simulink model "msk_sync"  (Simulink 6.0)
settings: Solver=FixedStepDiscrete  SolverMode=SingleTasking  StartTime=0.0  StopTime=2.0  RelTol=1e-3
PreLoadFcn:
  | warning off MATLAB:dispatcher:InexactMatch;
model workspace: external: M-Code (data not in the file)
undefined symbols (not defined in the file or in its folder): sampPerSymb, slcm, tsym
libraries: dspsrcs4 x9, simulink x5, commsink2 x4, dspsigops x4, commblksprivate x2, dspsigattribs x2, dspstat3 x2, commutil2 x2, commdigbbndcpm2 x2, dspobslib x1, commfilt2 x1, dspmathops x1
CloseFcn:
  | if exist('msk_sync_sigsOut','var'), clear msk_sync_sigsOut; end;
  | warning on MATLAB:dispatcher:InexactMatch;
settings Model: Creator=arodrigu  LastModifiedBy=cvora  ExtModeAutoUpdateStatusClock=off  ProdHWDeviceType=Specified
settings DataIOCC: LimitDataPoints=off  SaveOutput=off  SaveTime=off  SignalLoggingName=msk_sync_sigsOut
settings OptimizationCC: BooleanDataType=off
settings DebuggingCC: CheckExecutionContextPreStartOutputMsg=on  CheckExecutionContextRuntimeOutputMsg=on  SolverPrmCheckMsg=none  InheritedTsInSrcMsg=none
settings HardwareCC: ProdHWDeviceType=Specified
settings ModelReferenceCC: UpdateModelReferenceTargets=IfOutOfDate

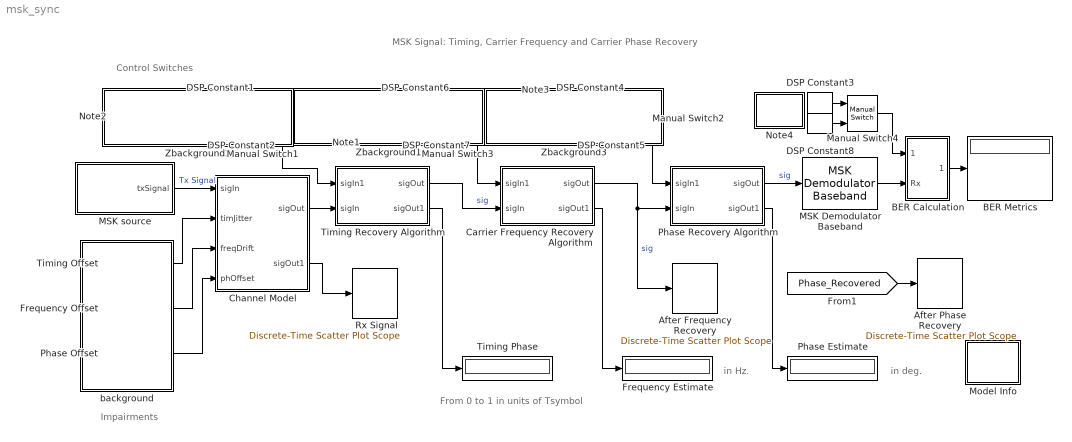
== system msk_sync ==
  note: MSK Signal:
      | Timing, Carrier Frequency and Carrier Phase Recovery
  note: in Hz.
  note: From 0 to 1
      | in units of Tsymbol
  note: in deg.
  note: Control Switches
  note: Impairments
  After Frequency Recovery : commsink2/Discrete-Time Scatter Plot Scope  Tag=ScatterPlot  sampPerSymb=1  offsetEye=0  numTraces=2000  numNewFrames=1000  LineMarkers=.  LineColors=b  fading=on  render=on  AxisGrid=on  xMin=-1.5  xMax=1.5  yMin=-1.5  yMax=1.5  inphaseLabel=In-phase Amplitude  quadratureLabel=Quadrature Amplitude  openScopeAtSimStart=on  FrameNumber=off  FigPos=[435 41 358 358]  figTitle=Scatter Plot  numLinesMax=8  block_type_=scatter
  After Phase Recovery : commsink2/Discrete-Time Scatter Plot Scope  Tag=ScatterPlot  sampPerSymb=1  offsetEye=0  numTraces=2000  numNewFrames=1000  LineMarkers=.  LineColors=b  fading=on  render=on  AxisGrid=on  xMin=-1.5  xMax=1.5  yMin=-1.5  yMax=1.5  inphaseLabel=In-phase Amplitude  quadratureLabel=Quadrature Amplitude  openScopeAtSimStart=on  FrameNumber=off  FigPos=[832 41 358 358]  figTitle=Scatter Plot  numLinesMax=8  block_type_=scatter
  BER Calculation : Subsystem  PropExecContextAcrossSSBoundary=on
      mask Display: disp('BER')
  BER Metrics : Display
  Carrier Frequency Recovery Algorithm : Subsystem  PropExecContextAcrossSSBoundary=on
      mask Type: Carrier Frequency Recovery algorithm
      mask Display: disp('Carrier Freq.\nRecovery')
  Channel Model : Subsystem  PropExecContextAcrossSSBoundary=on
      mask Type: RF Impairments
      mask Display:
      | plot(-10,-10,110, 110,[05 15 10 10 05 10 18 14 13 7.5 13 41 44 47 50 53 57
      | 59 100-[13 7.5 13 14 18 10 5 10 10 15 5]],[70 70 70 85 92 85 79 82 90 88.5
      | 90 90 87 93 87 93 87 90 90 88.5 90 82 79 85 92 85 70 70 70]-30);
  DSP Constant{1,3..4,6} (4 alike) : dspsrcs4/DSP Constant  Value=1  SampleMode=Discrete  discreteOutput=Sample-based (interpret vectors as 1-D)  continuousOutput=Sample-based  sampTime=tsym*1000  framePeriod=tsym*1000  dataType=Inherit from 'Constant value'  isSigned=on  wordLen=16  udDataType=sfix(16)  fracBitsMode=Best precision  numFracBits=15  InterpretAs1D=on  Ts=tsym*1000  FramebasedOutput=off
      settings: AttributesFormatString=\n\n\n\n
  DSP Constant{2,5,7..8} (4 alike) : dspsrcs4/DSP Constant  Value=0  SampleMode=Discrete  discreteOutput=Sample-based (interpret vectors as 1-D)  continuousOutput=Sample-based  sampTime=tsym*1000  framePeriod=tsym*1000  dataType=Inherit from 'Constant value'  isSigned=on  wordLen=16  udDataType=sfix(16)  fracBitsMode=Best precision  numFracBits=15  InterpretAs1D=on  Ts=tsym*1000  FramebasedOutput=off
      settings: AttributesFormatString=\n\n\n\n
  Frequency Estimate : Display
  Frequency Offset : Constant  Value=50
  MSK Demodulator Baseband : commdigbbndcpm2/MSK Demodulator Baseband  outputType=Bit  phaseOffset=0  samplesPerSymbol=1  traceBack=trDepth
  MSK source : Subsystem  PropExecContextAcrossSSBoundary=on
      mask Type: GMSK source
      mask Display: disp('MSK\nSource')
  Manual Switch1 : simulink/Signal Routing/Manual Switch  sw=1  action=0
  Manual Switch2 : simulink/Signal Routing/Manual Switch  sw=1  action=0
  Manual Switch3 : simulink/Signal Routing/Manual Switch  sw=1  action=0
  Manual Switch4 : simulink/Signal Routing/Manual Switch  sw=0  action=0
  Model Info : Subsystem  LoadFcn=slcm LoadBlock;  InitFcn=slcm('UpdateAllCMBlocksInThisModelInit')  PropExecContextAcrossSSBoundary=on  mask(CMBlock){InitialSaveTempField=, InitialBlockCM=None, BlockCM=None, Frame=on, SaveTempField=, DisplayStringWithTags=Info, MaskDisplayString=Info, HorizontalTextAlignment=Center, LeftAlignmentValue=0.5, SourceBlockDiagram=msk_sync, TagMaxNumber=20, CMTag1=, CMTag2=, CMTag3=, CMTag4=, CMTag5=, CMTag6=, CMTag7=, CMTag8=, CMTag9=, CMTag10=, CMTag11=, CMTag12=, CMTag13=, CMTag14=, CMTag15=, CMTag16=, CMTag17=, CMTag18=, CMTag19=, CMTag20=}
      mask help: This block allows revision control information to be displayed within the model.
      settings: CopyFcn=slcm CopyBlock;  DeleteFcn=slcm Cancel;  PostSaveFcn=slcm('UpdateAllCMBlocksInThisModel')  NameChangeFcn=slcm Rename;  OpenFcn=commdemohelp;
      mask Display: text(str2num(LeftAlignmentValue), 0.5, MaskDisplayString, 'HorizontalAlignment', HorizontalTextAlignment)
  Note1 : Subsystem  PropExecContextAcrossSSBoundary=on
      mask Display: disp('Carrier Frequency\nRecovery')
  Note2 : Subsystem  PropExecContextAcrossSSBoundary=on
      mask Display: disp('Timing Phase\nRecovery')
  Note3 : Subsystem  PropExecContextAcrossSSBoundary=on
      mask Display: disp('Phase\nRecovery')
  Note4 : Subsystem  PropExecContextAcrossSSBoundary=on
      mask Display: disp('Reset\nBER')
  Phase Estimate : Display
  Phase Offset : Constant  Value=30
  Phase Recovery Algorithm : Subsystem  PropExecContextAcrossSSBoundary=on
      mask Type: Carrier Frequency Recovery algorithm
      mask Display: disp('Phase\nRecovery')
  Rx Signal : commsink2/Discrete-Time Scatter Plot Scope  Tag=ScatterPlot  sampPerSymb=14  offsetEye=0  numTraces=2000  numNewFrames=1000  LineMarkers=.  LineColors=b  fading=on  render=on  AxisGrid=on  xMin=-1.5  xMax=1.5  yMin=-1.5  yMax=1.5  inphaseLabel=In-phase Amplitude  quadratureLabel=Quadrature Amplitude  openScopeAtSimStart=on  FrameNumber=off  FigPos=[38 41 358 358]  figTitle=Scatter Plot  numLinesMax=8  block_type_=scatter
  Timing Offset : Constant  Value=0.2
  Timing Phase : Display
  Timing Recovery Algorithm : Subsystem  PropExecContextAcrossSSBoundary=on
      mask Type: Timing recovery algorithm.
      mask Display: disp('Timing\nRecovery');
  Zbackground1 : Subsystem  PropExecContextAcrossSSBoundary=on
      mask Display: disp('')
  Zbackground2 : Subsystem  PropExecContextAcrossSSBoundary=on
      mask Display: disp('')
  Zbackground3 : Subsystem  PropExecContextAcrossSSBoundary=on
      mask Display: disp('')
  background : Subsystem  PropExecContextAcrossSSBoundary=on
      mask Display: disp('')
  wires:
  Carrier Frequency Recovery Algorithm/1(sigOut) -> Phase Recovery Algorithm/2(sigIn), After Frequency Recovery/1  "sig"
  MSK source/1(txSignal) -> Channel Model/1(sigIn)  "Tx Signal"
  Channel Model/1(sigOut) -> Timing Recovery Algorithm/2(sigIn)
  Manual Switch1/1 -> Timing Recovery Algorithm/1(sigIn1)
  Timing Recovery Algorithm/1(sigOut) -> Carrier Frequency Recovery Algorithm/2(sigIn)  "sig"
  Manual Switch3/1 -> Carrier Frequency Recovery Algorithm/1(sigIn1)
  Timing Offset/1 -> Channel Model/2(timJitter)
  Frequency Offset/1 -> Channel Model/3(freqDrift)
  Timing Recovery Algorithm/2(sigOut1) -> Timing Phase/1
  Carrier Frequency Recovery Algorithm/2(sigOut1) -> Frequency Estimate/1
  Phase Recovery Algorithm/2(sigOut1) -> Phase Estimate/1
  Phase Offset/1 -> Channel Model/4(phOffset)
  Phase Recovery Algorithm/1(sigOut) -> MSK Demodulator Baseband/1  "sig"
  MSK Demodulator Baseband/1 -> BER Calculation/2(Rx)
  BER Calculation/1(Out1) -> BER Metrics/1
  Channel Model/2(sigOut1) -> Rx Signal/1
  Manual Switch4/1 -> BER Calculation/1(Rst)
  [Phase_Recovered] -> After Phase Recovery/1
  Manual Switch2/1 -> Phase Recovery Algorithm/1(sigIn1)
  DSP Constant4/1 -> Manual Switch2/1
  DSP Constant5/1 -> Manual Switch2/2
  DSP Constant6/1 -> Manual Switch3/1
  DSP Constant7/1 -> Manual Switch3/2
  DSP Constant1/1 -> Manual Switch1/1
  DSP Constant2/1 -> Manual Switch1/2
  DSP Constant3/1 -> Manual Switch4/1
  DSP Constant8/1 -> Manual Switch4/2

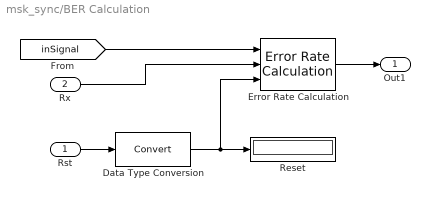
== system msk_sync/BER Calculation ==
  Rst : Inport  LatchInput=off
  Rx : Inport  Port=2  LatchInput=off
  Data Type Conversion : DataTypeConversion  OutDataTypeMode=double
  Error Rate Calculation : commsink2/Error Rate Calculation  N=trDepth+2 % Traceback Depth + Delay due to Timing Recovery  st_delay=0  cp_mode=Entire frame  subframe=[]  PMode=Port  WsName=ErrorVec  RsMode2=on  stop=off  numErr=100  maxBits=1e6
  Reset : Display
  Out1 : Outport
  wires:
  Error Rate Calculation/1 -> Out1/1
  Rst/1 -> Data Type Conversion/1
  Data Type Conversion/1 -> Reset/1, Error Rate Calculation/3
  Rx/1 -> Error Rate Calculation/2
  [inSignal] -> Error Rate Calculation/1

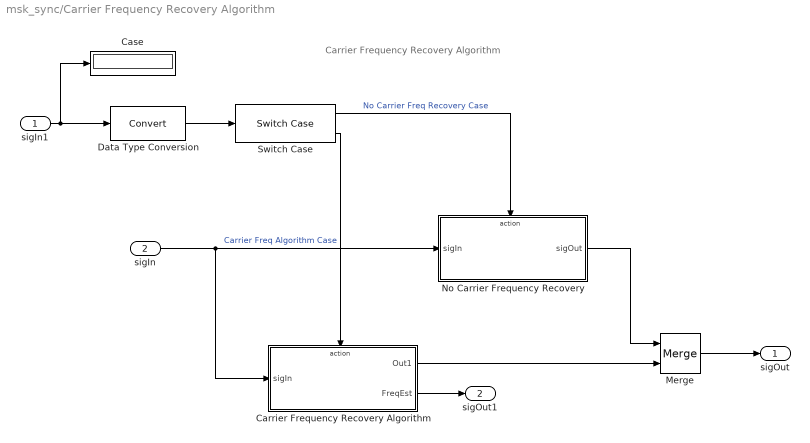
== system msk_sync/Carrier Frequency Recovery Algorithm ==
  note: Carrier Frequency Recovery Algorithm
  sigIn1 : Inport  LatchInput=off
  sigIn : Inport  Port=2  LatchInput=off
  Carrier Frequency Recovery Algorithm : Subsystem  TreatAsAtomicUnit=on  PropExecContextAcrossSSBoundary=on
  Case : Display
  Data Type Conversion : DataTypeConversion  OutDataTypeMode=double
  Merge : Merge
  No Carrier Frequency Recovery : Subsystem  TreatAsAtomicUnit=on  PropExecContextAcrossSSBoundary=on
  Switch Case : SwitchCase  CaseConditions={0,1}  CaseShowDefault=off
  sigOut : Outport
  sigOut1 : Outport  Port=2
  wires:
  sigIn/1 -> No Carrier Frequency Recovery/1(sigIn), Carrier Frequency Recovery Algorithm/1(sigIn)
  Merge/1 -> sigOut/1
  Switch Case/2 -> Carrier Frequency Recovery Algorithm/Action  "Carrier Freq Algorithm Case"
  Switch Case/1 -> No Carrier Frequency Recovery/Action  "No Carrier Freq Recovery Case"
  No Carrier Frequency Recovery/1(sigOut) -> Merge/1
  Carrier Frequency Recovery Algorithm/1(Out1) -> Merge/2
  Carrier Frequency Recovery Algorithm/2(FreqEst) -> sigOut1/1
  sigIn1/1 -> Data Type Conversion/1, Case/1
  Data Type Conversion/1 -> Switch Case/1

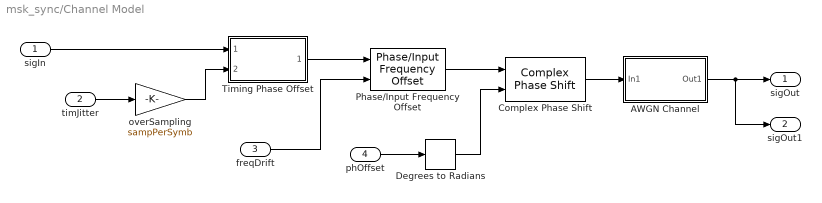
== system msk_sync/Channel Model ==
  sigIn : Inport  LatchInput=off
  timJitter : Inport  Port=2  LatchInput=off
  freqDrift : Inport  Port=3  LatchInput=off
  phOffset : Inport  Port=4  LatchInput=off
  AWGN Channel : Subsystem  AncestorBlock=commchan2/AWGN Channel  PropExecContextAcrossSSBoundary=on  mask(AWGN Channel){seed=67, noiseMode=Signal to noise ratio  (Eb/No), EbNodB=60, EsNodB=10, SNRdB=10, bitsPerSym=1, Ps=1, Tsym=tsym, variance=1}
      mask prompts: seed "Initial seed:"; noiseMode "Mode:"; EbNodB "Eb/No (dB):"; EsNodB "Es/No (dB):"; SNRdB "SNR (dB):"; bitsPerSym "Number of bits per symbol:"; Ps "Input signal power (watts):"; Tsym "Symbol period (s):"
      mask help:
      | Add white Gaussian noise to the input signal. The input and output signals can be real or complex. This block supports multichannel input and output signals as well as frame-based processing.
      |
      | When using either of the variance modes with complex inputs, the variance values are equally divided among the real and imaginary components of the input signal.
      mask init:
      | [mode,s]=commblkawgnchan2(gcb,'init');
      | if ~isempty(s.status) error(s.status); end
      mask Help: helpview(commbhelp)
      mask StyleString: edit,popup(Signal to noise ratio  (Eb/No)|Signal to noise ratio  (Es/No)|Signal to noise ratio  (SNR)|Variance from mask|Variance from port),edit,edit,edit,edit,edit,edit,edit
      mask CallbackString: |commblkawgnchan2(gcb,'Mode');|||||||
      mask Display:
      | plot(-10,-10,110, 110,[05 15 10 10 05 10 18 14 13 7.5 13 41 44 47 50 53 57
      | 59 100-[13 7.5 13 14 18 10 5 10 10 15 5]],[70 70 70 85 92 85 79 82 90 88.5
      | 90 90 87 93 87 93 87 90 90 88.5 90 82 79 85 92 85 70 70 70]);
      | disp('AWGN');
      | port_label('input',s.i1,s.i1s);
      | port_label('input',s.i2,s.i2s);
      | port_label('output',s.o1,s.o1s);
  Complex Phase Shift : commutil2/Complex Phase Shift
  Degrees to Radians : simulink_extras/Transformations/Degrees to Radians
  Phase/Input Frequency Offset : commblksprivate/Phase//Input Frequency Offset  phaseOffset=0
  Timing Phase Offset : Subsystem  PropExecContextAcrossSSBoundary=on
      mask Display: disp('Timing Phase\nOffset')
  overSampling : Gain  Gain=sampPerSymb  SaturateOnIntegerOverflow=on
  sigOut : Outport
  sigOut1 : Outport  Port=2
  wires:
  AWGN Channel/1(Out1) -> sigOut/1, sigOut1/1
  sigIn/1 -> Timing Phase Offset/1(InSignal)
  timJitter/1 -> overSampling/1
  Timing Phase Offset/1(OutSignal) -> Phase/Input Frequency Offset/1
  overSampling/1 -> Timing Phase Offset/2(phOffset)
  freqDrift/1 -> Phase/Input Frequency Offset/2
  Phase/Input Frequency Offset/1 -> Complex Phase Shift/1
  Complex Phase Shift/1 -> AWGN Channel/1(In1)
  Degrees to Radians/1 -> Complex Phase Shift/2
  phOffset/1 -> Degrees to Radians/1

== system msk_sync/MSK source ==
  note: in bps.
  Bernoulli Binary Generator : commrandsrc2/Bernoulli Binary Generator  P=0.5  seed=61  Ts=tsym  frameBased=on  sampPerFrame=1000  orient=off
  Compute Bit Rate : Subsystem  PropExecContextAcrossSSBoundary=on  mask(Compute bit rate of signal ){overSamp=sampPerSymb}
      mask prompts: overSamp "Oversampling factor:"
      mask help: Bit rate calculation based on probed sample time and a specified number of bits per sample.
      mask Display: disp('Compute\nBit Rate')
  MSK Modulator Baseband : commdigbbndcpm2/MSK Modulator Baseband  inputType=Bit  phaseOffset=0  samplesPerSymbol=sampPerSymb
  bit rate : Display
  txSignal : Outport
  tag scope: inSignal=global
  wires:
  Bernoulli Binary Generator/1 -> [inSignal], MSK Modulator Baseband/1
  MSK Modulator Baseband/1 -> Compute Bit Rate/1(sig), txSignal/1
  Compute Bit Rate/1(rate) -> bit rate/1

== system msk_sync/Model Info ==
  EmptySubsystem : Subsystem  PropExecContextAcrossSSBoundary=on

== system msk_sync/Note1 ==

== system msk_sync/Note2 ==

== system msk_sync/Note3 ==

== system msk_sync/Note4 ==

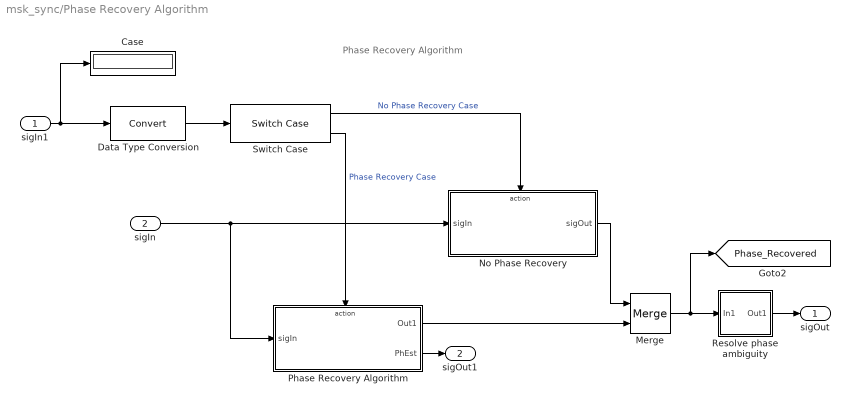
== system msk_sync/Phase Recovery Algorithm ==
  note: Phase Recovery Algorithm
  sigIn1 : Inport  LatchInput=off
  sigIn : Inport  Port=2  LatchInput=off
  Case : Display
  Data Type Conversion : DataTypeConversion  OutDataTypeMode=double
  Merge : Merge
  No Phase Recovery : Subsystem  TreatAsAtomicUnit=on  PropExecContextAcrossSSBoundary=on
  Phase Recovery Algorithm : Subsystem  TreatAsAtomicUnit=on  PropExecContextAcrossSSBoundary=on
  Resolve phase ambiguity : Subsystem  PropExecContextAcrossSSBoundary=on
  Switch Case : SwitchCase  CaseConditions={0,1}  CaseShowDefault=off
  sigOut : Outport
  sigOut1 : Outport  Port=2
  tag scope: Phase_Recovered=global
  wires:
  Data Type Conversion/1 -> Switch Case/1
  sigIn1/1 -> Case/1, Data Type Conversion/1
  Phase Recovery Algorithm/2(PhEst) -> sigOut1/1
  Phase Recovery Algorithm/1(Out1) -> Merge/2
  No Phase Recovery/1(sigOut) -> Merge/1
  Switch Case/1 -> No Phase Recovery/Action  "No Phase Recovery Case"
  Switch Case/2 -> Phase Recovery Algorithm/Action  "Phase Recovery Case"
  Merge/1 -> Resolve phase ambiguity/1(In1), [Phase_Recovered]
  sigIn/1 -> Phase Recovery Algorithm/1(sigIn), No Phase Recovery/1(sigIn)
  Resolve phase ambiguity/1(Out1) -> sigOut/1

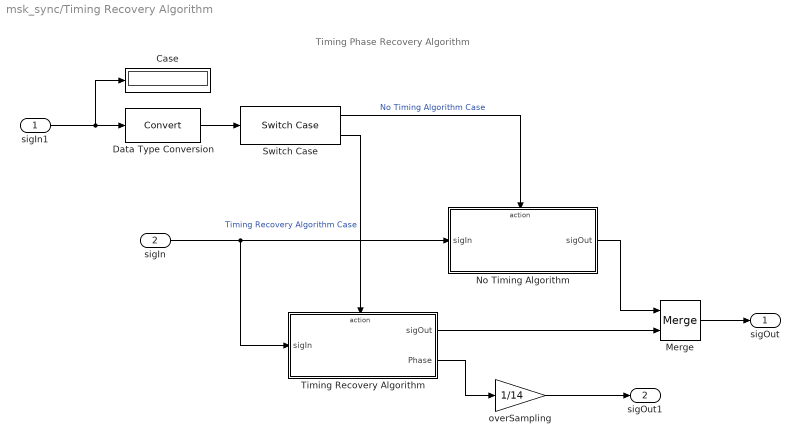
== system msk_sync/Timing Recovery Algorithm ==
  note: Timing Phase Recovery Algorithm
  sigIn1 : Inport  LatchInput=off
  sigIn : Inport  Port=2  LatchInput=off
  Case : Display
  Data Type Conversion : DataTypeConversion  OutDataTypeMode=double
  Merge : Merge
  No Timing Algorithm : Subsystem  TreatAsAtomicUnit=on  PropExecContextAcrossSSBoundary=on
  Switch Case : SwitchCase  CaseConditions={0,1}  CaseShowDefault=off
  Timing Recovery Algorithm : Subsystem  TreatAsAtomicUnit=on  PropExecContextAcrossSSBoundary=on
  overSampling : Gain  Gain=1/14  SaturateOnIntegerOverflow=on
  sigOut : Outport
  sigOut1 : Outport  Port=2
  wires:
  sigIn/1 -> Timing Recovery Algorithm/1(sigIn), No Timing Algorithm/1(sigIn)
  Merge/1 -> sigOut/1
  Switch Case/2 -> Timing Recovery Algorithm/Action  "Timing Recovery Algorithm Case"
  Switch Case/1 -> No Timing Algorithm/Action  "No Timing Algorithm Case"
  No Timing Algorithm/1(sigOut) -> Merge/1
  Timing Recovery Algorithm/1(sigOut) -> Merge/2
  Timing Recovery Algorithm/2(Phase) -> overSampling/1
  sigIn1/1 -> Data Type Conversion/1, Case/1
  overSampling/1 -> sigOut1/1
  Data Type Conversion/1 -> Switch Case/1

== system msk_sync/Zbackground1 ==
  note: This subsystem is empty

== system msk_sync/Zbackground2 ==
  note: This subsystem is empty

== system msk_sync/Zbackground3 ==
  note: This subsystem is empty

== system msk_sync/background ==
  note: This subsystem is empty

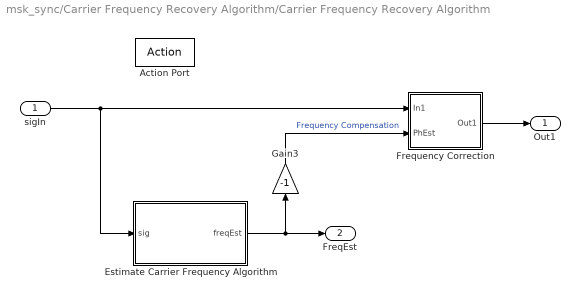
== system msk_sync/Carrier Frequency Recovery Algorithm/Carrier Frequency Recovery Algorithm ==
  sigIn : Inport  LatchInput=off
  Action Port : ActionPort  InitializeStates=reset  ActionType=case
  Estimate Carrier Frequency Algorithm : Subsystem  PropExecContextAcrossSSBoundary=on
  Frequency Correction : Subsystem  PropExecContextAcrossSSBoundary=on
      mask Display: disp('Frequency\nCorrection');
  Gain3 : Gain  Orientation=up  Gain=-1  SaturateOnIntegerOverflow=on
  Out1 : Outport
  FreqEst : Outport  Port=2  OutputWhenDisabled=reset  InitialOutput=0
  wires:
  sigIn/1 -> Estimate Carrier Frequency Algorithm/1(sig), Frequency Correction/1(In1)
  Frequency Correction/1(Out1) -> Out1/1
  Gain3/1 -> Frequency Correction/2(PhEst)  "Frequency Compensation"
  Estimate Carrier Frequency Algorithm/1(freqEst) -> FreqEst/1, Gain3/1

== system msk_sync/Carrier Frequency Recovery Algorithm/No Carrier Frequency Recovery ==
  sigIn : Inport  LatchInput=off
  Action Port : ActionPort  ActionType=case
  sigOut : Outport
  wires:
  sigIn/1 -> sigOut/1

== system msk_sync/Channel Model/AWGN Channel ==
  In1 : Inport  LatchInput=off
  Dynamic AWGN : S-Function  FunctionName=scomawgnchan2  Parameters=noiseMode, EbNodB, EsNodB, SNRdB, bitsPerSym, Ps, Tsym, variance
  Random Source : dspsrcs4/Random Source  SrcType=Gaussian  NormMethod=Ziggurat  CltLength=12  Min=0  Max=1  Mean=0  Var=1  RepMode=Specify seed  Seed=seed  Inherit=on  SampMode=Discrete  SampTime=1  SampFrame=1  DataType=Double  OutComplex=Real
  Variance : Ground
  Out1 : Outport
  wires:
  Variance/1 -> Dynamic AWGN/3
  Dynamic AWGN/1 -> Out1/1
  In1/1 -> Dynamic AWGN/1
  Random Source/1 -> Dynamic AWGN/2

== system msk_sync/Channel Model/Timing Phase Offset ==
  InSignal : Inport  LatchInput=off
  phOffset : Inport  Port=2  LatchInput=off
  Variable Fractional Delay : dspsigops/Variable Fractional Delay  mode=Linear Interpolation  dmax=100  L=4  R=10  alpha=1  ic=0
  OutSignal : Outport
  wires:
  Variable Fractional Delay/1 -> OutSignal/1
  InSignal/1 -> Variable Fractional Delay/1
  phOffset/1 -> Variable Fractional Delay/2

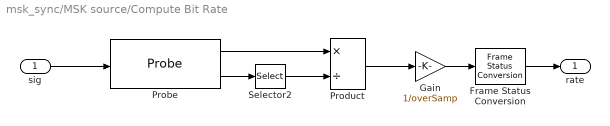
== system msk_sync/MSK source/Compute Bit Rate ==
  sig : Inport  LatchInput=off
  Frame Status Conversion : dspsigattribs/Frame Status Conversion  growRefPort=off  outframe=Frame-based
  Gain : Gain  Gain=1/overSamp  SaturateOnIntegerOverflow=on
  Probe : Probe  ProbeComplexSignal=off
  Product : Product  Inputs=*/  SaturateOnIntegerOverflow=on  InputSameDT=on
  Selector2 : Selector  Elements=[1 ]  InputPortWidth=2
  rate : Outport
  wires:
  Product/1 -> Gain/1
  sig/1 -> Probe/1
  Selector2/1 -> Product/2
  Probe/2 -> Selector2/1
  Probe/1 -> Product/1
  Gain/1 -> Frame Status Conversion/1
  Frame Status Conversion/1 -> rate/1

== system msk_sync/Model Info/EmptySubsystem ==

== system msk_sync/Phase Recovery Algorithm/No Phase Recovery ==
  sigIn : Inport  LatchInput=off
  Action Port : ActionPort  ActionType=case
  sigOut : Outport
  wires:
  sigIn/1 -> sigOut/1

== system msk_sync/Phase Recovery Algorithm/Phase Recovery Algorithm ==
  sigIn : Inport  LatchInput=off
  Action Port : ActionPort  InitializeStates=reset  ActionType=case
  CPM Phase Recovery : commphrec2/CPM Phase Recovery  P=2  intPeriod=1000
  Out1 : Outport
  PhEst : Outport  Port=2  OutputWhenDisabled=reset  InitialOutput=0
  wires:
  sigIn/1 -> CPM Phase Recovery/1
  CPM Phase Recovery/1 -> Out1/1
  CPM Phase Recovery/2 -> PhEst/1

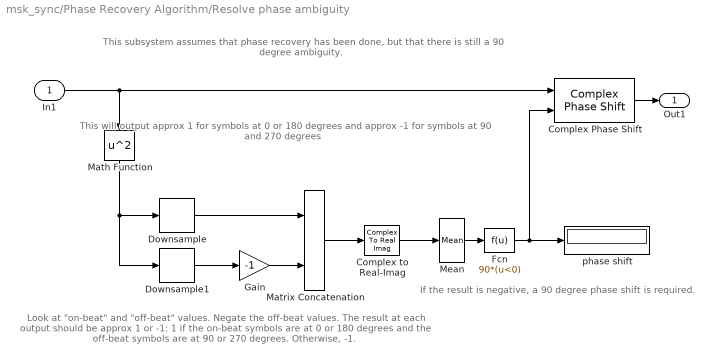
== system msk_sync/Phase Recovery Algorithm/Resolve phase ambiguity ==
  note: If the result is negative,
      | a 90 degree phase shift is required.
  note: Look at "on-beat" and "off-beat" values.
      | Negate the off-beat values.
      | The result at each output should be approx 1 or -1:
      | 1 if the on-beat symbols are at 0 or 180 degrees
      | and the off-beat symbols are at 90 or 270 degrees.
      | Otherwise, -1.
  note: This will output approx 1 for symbols at 0 or 180 degrees
      | and approx -1 for symbols at 90 and 270 degrees
  note: This subsystem assumes that phase recovery has been done, but that there is still a 90 degree ambiguity.
  In1 : Inport  LatchInput=off
  Complex Phase Shift : commutil2/Complex Phase Shift
  Complex to Real-Imag : ComplexToRealImag  Output=Real
  Downsample : dspsigops/Downsample  N=2  phase=0  ic=0  smode=Allow multirate  fmode=Maintain input frame rate
  Downsample1 : dspsigops/Downsample  N=2  phase=1  ic=0  smode=Allow multirate  fmode=Maintain input frame rate
  Fcn : Fcn  Expr=90*(u<0)
  Gain : Gain  Gain=-1
  Math Function : Math  Orientation=down  Operator=square  SaturateOnIntegerOverflow=on
  Matrix Concatenation : simulink/Math Operations/Matrix Concatenation  numInports=2  catMethod=Vertical
  Mean : dspstat3/Mean  run=off  reset_popup=None  roundingMode=Floor  overflowMode=off
  phase shift : Display
  Out1 : Outport
  wires:
  Fcn/1 -> Complex Phase Shift/2, phase shift/1
  Complex to Real-Imag/1 -> Mean/1
  Mean/1 -> Fcn/1
  Matrix Concatenation/1 -> Complex to Real-Imag/1
  Gain/1 -> Matrix Concatenation/2
  Downsample1/1 -> Gain/1
  Downsample/1 -> Matrix Concatenation/1
  Math Function/1 -> Downsample1/1, Downsample/1
  Complex Phase Shift/1 -> Out1/1
  In1/1 -> Math Function/1, Complex Phase Shift/1

== system msk_sync/Timing Recovery Algorithm/No Timing Algorithm ==
  sigIn : Inport  LatchInput=off
  Action Port : ActionPort  ActionType=case
  Downsample : dspsigops/Downsample  N=14  phase=0  ic=0  smode=Allow multirate  fmode=Maintain input frame rate
  sigOut : Outport
  wires:
  sigIn/1 -> Downsample/1
  Downsample/1 -> sigOut/1

== system msk_sync/Timing Recovery Algorithm/Timing Recovery Algorithm ==
  note: The Sym output is the result of applying the
      | estimated phase correction to the input signal.
  note: The Ph output gives the phase estimate
      | for each symbol in the input signal.
  sigIn : Inport  LatchInput=off
  Action Port : ActionPort  InitializeStates=reset  ActionType=case
  MSK-Type Signal Timing Recovery : commtimrec2/MSK-Type Signal Timing Recovery  modType=MSK  sampPerSymbol=sampPerSymb  propGain=0.2  resetMode=None
  Multiport Selector : dspindex/Multiport Selector  rowsOrCols=Rows  idxCellArray={1}  idxErrMode=Clip Index
  sigOut : Outport
  Phase : Outport  Port=2  OutputWhenDisabled=reset  InitialOutput=0
  wires:
  sigIn/1 -> MSK-Type Signal Timing Recovery/1
  MSK-Type Signal Timing Recovery/1 -> sigOut/1
  MSK-Type Signal Timing Recovery/2 -> Multiport Selector/1
  Multiport Selector/1 -> Phase/1

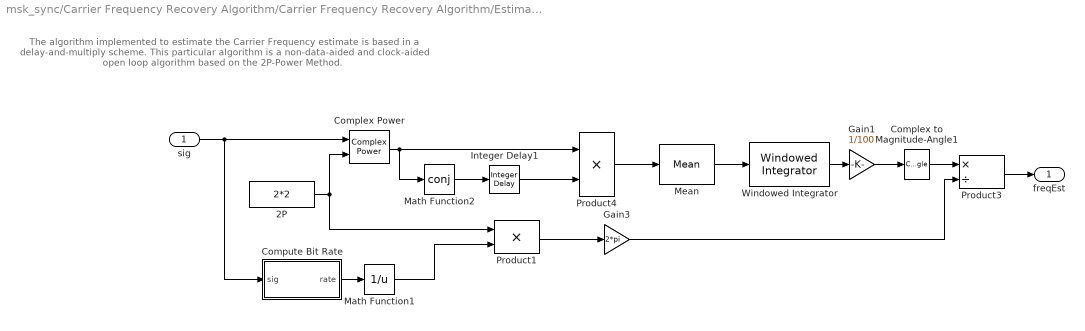
== system msk_sync/Carrier Frequency Recovery Algorithm/Carrier Frequency Recovery Algorithm/Estimate Carrier Frequency Algorithm ==
  note: The algorithm implemented to estimate the Carrier Frequency estimate is based in a
      | delay-and-multiply scheme. This particular algorithm is a non-data-aided
      | and clock-aided open loop algorithm based on the 2P-Power Method.
  sig : Inport  LatchInput=off
  2P : Constant  Value=2*2
  Complex Power : commblksprivate/Complex Power
  Complex to Magnitude-Angle1 : ComplexToMagnitudeAngle  Output=Angle
  Compute Bit Rate : Subsystem  PropExecContextAcrossSSBoundary=on  mask(Compute bit rate of signal ){overSamp=1}
      mask prompts: overSamp "Oversampling factor:"
      mask help: Bit rate calculation based on probed sample time and a specified number of bits per sample.
      mask Display: disp('Compute\nBit Rate')
  Gain1 : Gain  Gain=1/100  SaturateOnIntegerOverflow=on
  Gain3 : Gain  Gain=2*pi  SaturateOnIntegerOverflow=on
  Integer Delay1 : dspobslib/Integer Delay  delay=1  ic=1  reset_popup=None
  Math Function1 : Math  Operator=reciprocal  SaturateOnIntegerOverflow=on
  Math Function2 : Math  Operator=conj  SaturateOnIntegerOverflow=on
  Mean : dspstat3/Mean  run=off  reset_popup=None  roundingMode=Floor  overflowMode=off
  Product1 : Product  Inputs=**  SaturateOnIntegerOverflow=on
  Product3 : Product  Inputs=*/  SaturateOnIntegerOverflow=on
  Product4 : Product  SaturateOnIntegerOverflow=on
  Windowed Integrator : commfilt2/Windowed Integrator  integperiod=100
  freqEst : Outport
  wires:
  Product1/1 -> Gain3/1
  2P/1 -> Product1/1, Complex Power/2
  Complex Power/1 -> Product4/1, Math Function2/1
  Math Function2/1 -> Integer Delay1/1
  Integer Delay1/1 -> Product4/2
  Product4/1 -> Mean/1
  Complex to Magnitude-Angle1/1 -> Product3/1
  Gain3/1 -> Product3/2
  sig/1 -> Compute Bit Rate/1(sig), Complex Power/1
  Product3/1 -> freqEst/1
  Mean/1 -> Windowed Integrator/1
  Compute Bit Rate/1(rate) -> Math Function1/1
  Math Function1/1 -> Product1/2
  Gain1/1 -> Complex to Magnitude-Angle1/1
  Windowed Integrator/1 -> Gain1/1

== system msk_sync/Carrier Frequency Recovery Algorithm/Carrier Frequency Recovery Algorithm/Frequency Correction ==
  In1 : Inport  LatchInput=off
  PhEst : Inport  Port=2  LatchInput=off
  Calculate Frequency Offset : Subsystem  PropExecContextAcrossSSBoundary=on
      mask Display: disp('Calculate\nFrequency\nOffset');
  Product : Product  SaturateOnIntegerOverflow=on  InputSameDT=on
  Out1 : Outport
  wires:
  Calculate Frequency Offset/1(Out1) -> Product/2
  In1/1 -> Calculate Frequency Offset/1(In1), Product/1
  Product/1 -> Out1/1
  PhEst/1 -> Calculate Frequency Offset/2(Freq)

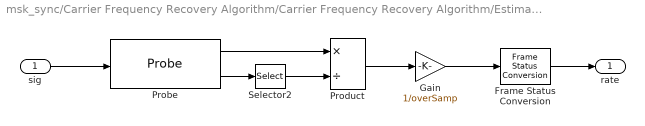
== system msk_sync/Carrier Frequency Recovery Algorithm/Carrier Frequency Recovery Algorithm/Estimate Carrier Frequency Algorithm/Compute Bit Rate ==
  sig : Inport  LatchInput=off
  Frame Status Conversion : dspsigattribs/Frame Status Conversion  growRefPort=off  outframe=Frame-based
  Gain : Gain  Gain=1/overSamp  SaturateOnIntegerOverflow=on
  Probe : Probe  ProbeComplexSignal=off
  Product : Product  Inputs=*/  SaturateOnIntegerOverflow=on  InputSameDT=on
  Selector2 : Selector  Elements=[1 ]  InputPortWidth=2
  rate : Outport
  wires:
  Product/1 -> Gain/1
  sig/1 -> Probe/1
  Selector2/1 -> Product/2
  Probe/2 -> Selector2/1
  Probe/1 -> Product/1
  Gain/1 -> Frame Status Conversion/1
  Frame Status Conversion/1 -> rate/1

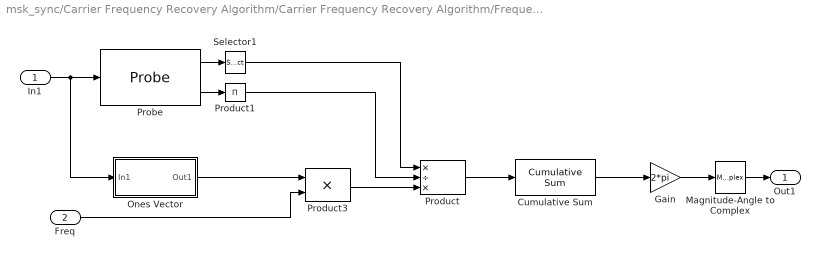
== system msk_sync/Carrier Frequency Recovery Algorithm/Carrier Frequency Recovery Algorithm/Frequency Correction/Calculate Frequency Offset ==
  In1 : Inport  LatchInput=off
  Freq : Inport  Port=2  LatchInput=off
  Cumulative Sum : dspmathops/Cumulative Sum  dim=Channels (running sum)  reset_popup=None
  Gain : Gain  Gain=2*pi  SaturateOnIntegerOverflow=on
  Magnitude-Angle to Complex : MagnitudeAngleToComplex  Input=Angle  ConstantPart=1
  Ones Vector : Subsystem  PropExecContextAcrossSSBoundary=on
      mask Type: Ones Vector
      mask Description: Create a vector of equals whose length is equal to input portwidth.
      mask Display: disp('Ones(1:length)')
  Probe : Probe  ProbeWidth=off  ProbeComplexSignal=off  ProbeSignalDimensions=on
  Product : Product  Inputs=*/*  SaturateOnIntegerOverflow=on  InputSameDT=on
  Product1 : Product  Inputs=1  SaturateOnIntegerOverflow=on  InputSameDT=on
  Product3 : Product  Inputs=**  SaturateOnIntegerOverflow=on
  Selector1 : Selector  Elements=[1 ]  InputPortWidth=2
  Out1 : Outport
  wires:
  Selector1/1 -> Product/1
  Product1/1 -> Product/2
  Probe/1 -> Selector1/1
  Product/1 -> Cumulative Sum/1
  Probe/2 -> Product1/1
  In1/1 -> Probe/1, Ones Vector/1(In1)
  Magnitude-Angle to Complex/1 -> Out1/1
  Gain/1 -> Magnitude-Angle to Complex/1
  Product3/1 -> Product/3
  Freq/1 -> Product3/2
  Cumulative Sum/1 -> Gain/1
  Ones Vector/1(Out1) -> Product3/1

== system msk_sync/Carrier Frequency Recovery Algorithm/Carrier Frequency Recovery Algorithm/Frequency Correction/Calculate Frequency Offset/Ones Vector ==
  In1 : Inport  LatchInput=off
  Bias : Bias  Bias=1
  Complex to Real-Imag : ComplexToRealImag  Output=Real
  Gain1 : Gain  Gain=0
  Out1 : Outport
  wires:
  Complex to Real-Imag/1 -> Gain1/1
  Gain1/1 -> Bias/1
  In1/1 -> Complex to Real-Imag/1
  Bias/1 -> Out1/1
